simulink model "modello_completo_simulink2019"  (R2019b)
settings: Solver=VariableStepAuto  StartTime=0.0  StopTime=10  RelTol=1e-3
values from neighbouring files (symbols this model uses):
  a = 0.35    [data.m]    (also in geodetic2nedS.m = 6378137)
  a1 = rho * D^4 * alpha1    (= 0.000388302366464)    [data.m]
  a2 = -rho * D^3 * alpha2 * (1 - omega)    (= 0.0037030698432)    [data.m]
  AHRS_bias = [0 0 0]    [data.m]
  AHRS_sample_time = 1/50    (= 0.02)    [data.m]
  AHRS_var = ([1 1 2] * pi/180).^2    [data.m]
  alpha1 = 0.0113    [data.m]
  alpha2 = -0.0091    [data.m]
  c = son2(1)    [Sonar_id.m]    (also in data.m = 0.19)
  current = [seaCurrent; 0; 0; 0]    [data.m]
  D = 0.076    [data.m]
  dead_zone_limit = 31.5    [data.m]
  DVL_sample_t = 1/12    (= 0.0833333333333)    [data.m]
  DVL_var1 = 0.005^2    (= 2.5e-05)    [data.m]
  DVL_var2 = 0.015^2    (= 0.000225)    [data.m]
  DVL_var3 = 0.023^2    (= 0.000529)    [data.m]
  gps_sample_t = 1    [data.m]
  H = eye(3)    [data.m]    (also in navigation_data.m)
  IMU_sample_time = 1/100    (= 0.01)    [data.m]
  initial = []    [data.m]
  INSP = unicode2native(inspectionDirection)    [data.m]
  Ki_bodypos1 = 0    [parametri_PID.m]
  Ki_bodypos2 = 0    [parametri_PID.m]
  Ki_bodypos3 = 0    [parametri_PID.m]
  Ki_bodypos4 = 0    [parametri_PID.m]
  Ki_bodypos5 = 0    [parametri_PID.m]
  Ki_depth1 = 0    [parametri_PID.m]
  Ki_depth2 = 0    [parametri_PID.m]
  Ki_depth3 = 0    [parametri_PID.m]
  Ki_depth4 = 0    [parametri_PID.m]
  Ki_depth5 = 0    [parametri_PID.m]
  Ki_latvel1 = 0    [parametri_PID.m]
  Ki_latvel2 = 0    [parametri_PID.m]
  Ki_latvel3 = 0    [parametri_PID.m]
  Ki_latvel4 = 0    [parametri_PID.m]
  Ki_latvel5 = 0    [parametri_PID.m]
  Ki_P1 = 0    [parametri_PID.m]
  Ki_P2 = 0    [parametri_PID.m]
  Ki_P3 = 0    [parametri_PID.m]
  Ki_P4 = 0    [parametri_PID.m]
  Ki_P5 = 0    [parametri_PID.m]
  Ki_R1 = 0    [parametri_PID.m]
  Ki_R2 = 0    [parametri_PID.m]
  Ki_R3 = 0    [parametri_PID.m]
  Ki_R4 = 0    [parametri_PID.m]
  Ki_R5 = 0    [parametri_PID.m]
  Ki_rel_or1 = 0    [parametri_PID.m]
  Ki_rel_or2 = 0    [parametri_PID.m]
  Ki_rel_or3 = 0    [parametri_PID.m]
  Ki_rel_or4 = 0    [parametri_PID.m]
  Ki_rel_or5 = 0    [parametri_PID.m]
  Ki_reldist1 = 0    [parametri_PID.m]
  Ki_reldist2 = 0    [parametri_PID.m]
  Ki_reldist3 = 0    [parametri_PID.m]
  Ki_reldist4 = 0    [parametri_PID.m]
  Ki_reldist5 = 0    [parametri_PID.m]
  Ki_surge1 = 0    [parametri_PID.m]
  Ki_surge2 = 0    [parametri_PID.m]
  Ki_surge3 = 0    [parametri_PID.m]
  Ki_surge4 = 0    [parametri_PID.m]
  Ki_surge5 = 0    [parametri_PID.m]
  Ki_yaw1 = 0    [parametri_PID.m]
  Ki_yaw2 = 0    [parametri_PID.m]
  Ki_yaw3 = 0    [parametri_PID.m]
  Ki_yaw4 = 0    [parametri_PID.m]
  Ki_yaw5 = 0    [parametri_PID.m]
  Kp_bodypos1 = 0    [parametri_PID.m]
  Kp_bodypos2 = 2    [parametri_PID.m]
  Kp_bodypos3 = 2    [parametri_PID.m]
  Kp_bodypos4 = 2    [parametri_PID.m]
  Kp_bodypos5 = 2    [parametri_PID.m]
  Kp_depth1 = 0    [parametri_PID.m]
  Kp_depth2 = 2    [parametri_PID.m]
  Kp_depth3 = 2    [parametri_PID.m]
  Kp_depth4 = 2    [parametri_PID.m]
  Kp_depth5 = 2    [parametri_PID.m]
  Kp_latvel1 = 0    [parametri_PID.m]
  Kp_latvel2 = 2    [parametri_PID.m]
  Kp_latvel3 = 2    [parametri_PID.m]
  Kp_latvel4 = 2    [parametri_PID.m]
  Kp_latvel5 = 2    [parametri_PID.m]
  Kp_P1 = 0    [parametri_PID.m]
  Kp_P2 = 2    [parametri_PID.m]
  Kp_P3 = 2    [parametri_PID.m]
  Kp_P4 = 2    [parametri_PID.m]
  Kp_P5 = 2    [parametri_PID.m]
  Kp_R1 = 0    [parametri_PID.m]
  Kp_R2 = 2    [parametri_PID.m]
  Kp_R3 = 2    [parametri_PID.m]
  Kp_R4 = 2    [parametri_PID.m]
  Kp_R5 = 2    [parametri_PID.m]
  Kp_rel_or1 = 0    [parametri_PID.m]
  Kp_rel_or2 = 2    [parametri_PID.m]
  Kp_rel_or3 = 2    [parametri_PID.m]
  Kp_rel_or4 = 2    [parametri_PID.m]
  Kp_rel_or5 = 2    [parametri_PID.m]
  Kp_reldist1 = 0    [parametri_PID.m]
  Kp_reldist2 = 2    [parametri_PID.m]
  Kp_reldist3 = 2    [parametri_PID.m]
  Kp_reldist4 = 2    [parametri_PID.m]
  Kp_reldist5 = 2    [parametri_PID.m]
  Kp_surge1 = 0    [parametri_PID.m]
  Kp_surge2 = 2    [parametri_PID.m]
  Kp_surge3 = 2    [parametri_PID.m]
  Kp_surge4 = 2    [parametri_PID.m]
  Kp_surge5 = 2    [parametri_PID.m]
  Kp_yaw1 = 0.6*6    (= 3.6)    [parametri_PID.m]
  Kp_yaw2 = 2    [parametri_PID.m]
  Kp_yaw3 = 2    [parametri_PID.m]
  Kp_yaw4 = 2    [parametri_PID.m]
  Kp_yaw5 = 2    [parametri_PID.m]
  M = M_rb + M_a    [Masse.m]
  M_inv = inv(M)    [Masse.m]
  n_max = 340    [data.m]
  num_cycle = 5    [data.m]    (also in navigation_data.m)
  omega = 0.1    [data.m]
  plot_smpl = 0.1    [data.m]
  ps_sample_t = 0.02    [data.m]
  ps_var = (5000/3)^2    (= 2777777.77778)    [data.m]
  pylonCenter = [ 43.723046 ... (first row only)    [missionB.m]
  ... (+4 more)
undefined symbols (not defined in the file or in its folder): DiscIntNeverNeededParam, s_data
libraries: simulink x3
(part 6 of 6)

== matlab function modello_completo_simulink2019/Controller/wrapTopi1 ==
  data: u input; y output
function y = fcn(u)
coder.extrinsic('wrapToPi');
y=0;
y = wrapToPi(u);
end

== matlab function modello_completo_simulink2019/Navigation1/Relative estimation/flag_sonar_func ==
  data: flag_sonar input; flag output; s_data parameter
function flag = fcn(flag_sonar, s_data)

flag = 1;

if sum(flag_sonar) >= (s_data.num-1)*8
    flag = 0;
else 
    flag = 1;
end

== matlab function modello_completo_simulink2019/Env. & Sensor Model1/DVL SENSOR/MATLAB Function2 ==
  data: v input; flag output
function flag  = vel_module(v)
%Calcola il modulo della velocità per controllare le condizioni di
%funzionamento del DVL

mod = sqrt((v(1))^2+(v(2))^2+(v(3))^2);

%Da datasheet, se la velocità è superiore ai 9 m/s il sensore non funziona bene
if mod > 9
    flag = 0;
else
    flag = 1;
end
end

== matlab function modello_completo_simulink2019/Env. & Sensor Model1/GPS SENSOR/NED2Geodetic ==
  data: depth input; u input; data_GDT output; enableGps input; pylonCenter parameter
%% Cast coordinates
% From NED (in m) to geodetic (in deg)
% If the gps is below of surface of the water they send 'NaN'
%
function data_GDT= fcn(depth, u, enableGps, pylonCenter)

lat_origin = pylonCenter(1);                                               % pylon is the center of the reference system
lon_origin = pylonCenter(2);
h_origin = pylonCenter(3);

xNorth = u(1);
yEast = u(2);

if enableGps == 1
    [lat,lon, h] = ned2geodeticS(xNorth, yEast, depth, lat_origin, lon_origin, h_origin);
else
    lat = NaN;
    lon = NaN;
end

data_GDT = [lat, lon];                                                     % Lat and lon are in degrees

== matlab function modello_completo_simulink2019/Env. & Sensor Model1/GPS SENSOR/Threshold ==
  data: depth output; x_out output; x_in input; y_out output; y_in input; h_in input; flag_enable_gps output; gpsThreshold parameter
%% Determines the exit flag based on depth
%
function [depth, x_out, y_out, flag_enable_gps] = fcn(x_in, y_in, h_in, gpsThreshold)


if (h_in > gpsThreshold)                                                   % gps does not work
    flag_enable_gps = 0;                                                   % because is below the surface of the water
    x_in = NaN;
    y_in = NaN;
else                                                                       % ok, gps work 
    flag_enable_gps = 1;
end

x_out = x_in;
y_out = y_in;
depth = h_in;

== matlab function modello_completo_simulink2019/Env. & Sensor Model1/Pressure sensor/MATLAB Function2 ==
  data: h input; p output; rho parameter
function p = pressure(h, rho)
%Calcola la pressione a partire dalla profondità

g = 9.81;                        %accelerazione gravitazionale
p = rho*g*h;
end

== matlab function modello_completo_simulink2019/Env. & Sensor Model1/Pressure sensor/MATLAB Function3 ==
  data: orient input; p input; h output; rho parameter; c parameter
function h = depth( orient,  p, rho, c)
%Calcola la profondità misurata dal sensore

phi = orient(1);
theta = orient(2);
psi = orient(3);
Rx_phi = [1 0 0; 0 cos(phi) -sin(phi); 0 sin(phi) cos(phi)];
Ry_theta = [cos(theta) 0 sin(theta); 0 1 0; -sin(theta) 0 cos(theta)];
Rz_psi = [cos(psi) -sin(psi) 0; sin(psi) cos(psi) 0; 0 0 1];

R = Rz_psi*Ry_theta*Rx_phi;
g = 9.81;
cNED = R*[0;0;c];                            %Vettore posizione dell'AUV in terna body riportato in terna NED
h = p/(rho*g)+cNED(3);                       %Il profondimetro è installato sulla pancia dell'AUV, lungo l'asse z
end

== matlab function modello_completo_simulink2019/Env. & Sensor Model1/Sonar sensor/MATLAB Function1 ==
  data: s_in input; s_out output; depth input; error input; flag output; s_data parameter
function [s_out,flag] = Sonar_lim(s_in,depth,error,s_data)
%SONAR_lim
%     [s_out,flag] = Sonar_id[s,error]
%
% Returns the sonar output considering the sensors limitations, but not
% taking into account the bias and error.
%
% flag signals that the corresponding sensor output is affected by
% problems:
% flag += 0     ==>     No errors
% flag += 1     ==>     Under minimum detectable range
% flag += 2     ==>     Over maximum detectable range
% flag += 4     ==>     Over maximum depth
% flag += 8     ==>     Other errors
%
% error is a boolean variable which, when true, sets the flag to += 8

s_data.num = 5;

flag = zeros(s_data.num,1);

s_out = s_in;

for i=1:s_data.num
    if s_in(i) < s_data.minrng
    % Too close
        flag(i) = flag(i)+1;
        s_out(i) = s_data.minrng;
    end
    
    if ( s_in(i) > s_data.maxrng || isnan(s_in(i)) )
    % Too far
        flag(i) = flag(i)+2;
        s_out(i) = NaN;
    end
    
    if depth > s_data.maxdpt
    % Over max depth
        flag(i) = flag(i)+4;
        s_out(i) = NaN;
    end
    
    if error(i) > 0
    % General error flag
        flag(i) = flag(i) + error(i);
        s_out(i) = NaN;
    end
end

end

== matlab function modello_completo_simulink2019/Env. & Sensor Model1/geodetic2NED1 ==
  data: x output; u input; y output; z output; pylonCenter parameter
%% Cast coordinates
% From deodetic (in deg) to NED (to m)
%
function [x, y, z] = fcn(u, pylonCenter)

lat_origin = pylonCenter(1);                                               % pylon is the center of the reference system
lon_origin= pylonCenter(2);
h_origin = pylonCenter(3);

lat = u(1);
lon = u(2);
h = u(3);


[xNorth, yEast, zDown] = geodetic2nedS(lat, lon, h, lat_origin, lon_origin, h_origin);

x = xNorth;                                                                % [m]
y = yEast;                                                                 % [m]
z = h;                                                                     % [m]
